simulink model "paper"  (R2022a)
settings: Solver=VariableStepAuto  StartTime=0.0  StopTime=10.0  RelTol=1e-3
values from neighbouring files (symbols this model uses):
  Ce = 0.556    [Untitled.m]    (also in liner.m)
  Ied = 4    [liner.m]
  Ki = 5    [Untitled.m]    (also in liner.m = 1)
  Kn = 7.84    [Untitled.m]    (also in liner.m = 29.75)
  Ks = 1    [Untitled.m]    (also in liner.m)
  ned = 5    [liner.m]
  R = 0.6    [Untitled.m]    (also in liner.m)
  Tl = 0.167    [Untitled.m]    (also in liner.m)
  Tm = 0.282    [Untitled.m]    (also in liner.m)
  Ts = 0.01    [Untitled.m]    (also in liner.m)
undefined symbols (not defined in the file or in its folder): alpha, beta, lambda, tau_i, tau_n, Ud, Ued
settings Model: Creator=houtonglei  LastModifiedBy=houtonglei
settings DataIOCC: SaveFinalState=on  SaveState=on

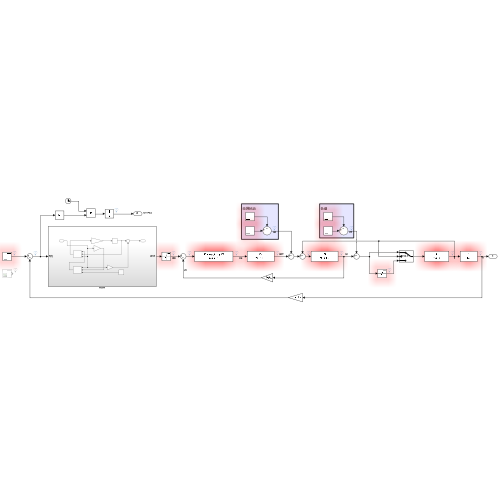
[thumbnail: Simulink's stored preview of the top-level diagram]
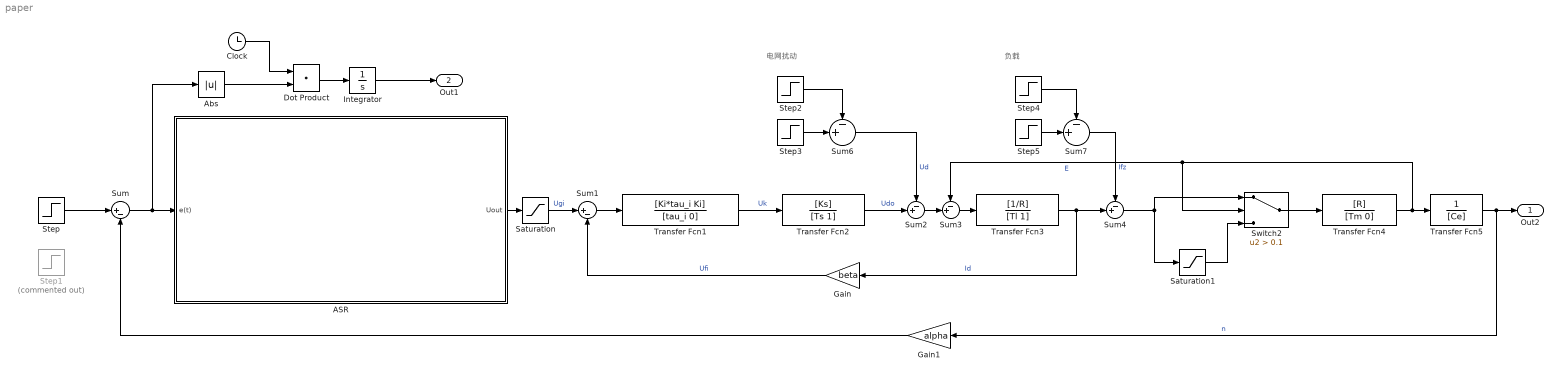
== system paper ==
  note: 负载
  note: 电网扰动
  ASR : Subsystem
  Abs : Abs  SaturateOnIntegerOverflow=off
  Clock : Clock
  Dot Product : DotProduct  OutDataTypeStr=Inherit: Inherit via internal rule
  Gain : Gain  Gain=beta
  Gain1 : Gain  Gain=alpha
  Integrator : Integrator
  Saturation : Saturate  UpperLimit=lambda*Ued  LowerLimit=-lambda*Ued
  Saturation1 : Saturate  UpperLimit=lambda*Ied  LowerLimit=0
  Step : Step  Time=0  After=ned  SampleTime=0
  Step1 : Step  Commented=on  Time=0  After=ned  SampleTime=0
  Step2 : Step  Time=2  After=-0.1*Ud  SampleTime=0
  Step3 : Step  After=-0.1*Ud  SampleTime=0
  Step4 : Step  Time=2  After=0.5*Ied  SampleTime=0
  Step5 : Step  After=0.5*Ied  SampleTime=0
  Sum : Sum  Inputs=|+-
  Sum1 : Sum  Inputs=|+-
  Sum{2..4,6..7} (5 alike) : Sum  Inputs=-+|
  Switch2 : Switch  Criteria=u2 > Threshold  Threshold=0.1  SaturateOnIntegerOverflow=off  InputSameDT=off
  Transfer Fcn1 : TransferFcn  Numerator=[Ki*tau_i Ki]  Denominator=[tau_i 0]  ContinuousStateAttributes='ACR'
  Transfer Fcn2 : TransferFcn  Numerator=[Ks]  Denominator=[Ts 1]  ContinuousStateAttributes='PWM'
  Transfer Fcn3 : TransferFcn  Numerator=[1/R]  Denominator=[Tl 1]
  Transfer Fcn4 : TransferFcn  Numerator=[R]  Denominator=[Tm 0]
  Transfer Fcn5 : TransferFcn  Denominator=[Ce]
  Out2 : Outport
  Out1 : Outport  Port=2  SignalName=J(ITAE)
  wires:
  Saturation/1 -> Sum1/1  "Ugi"
  Gain1/1 -> Sum/2
  Gain/1 -> Sum1/2  "Ufi"
  Transfer Fcn1/1 -> Transfer Fcn2/1  "Uk"
  Sum2/1 -> Sum3/2
  Transfer Fcn4/1 -> Transfer Fcn5/1, Switch2/2, Sum3/1  "E"
  Transfer Fcn5/1 -> Out2/1, Gain1/1  "n"
  Transfer Fcn2/1 -> Sum2/2  "Udo"
  Clock/1 -> Dot Product/1
  Abs/1 -> Dot Product/2
  Dot Product/1 -> Integrator/1
  Sum3/1 -> Transfer Fcn3/1
  Integrator/1 -> Out1/1
  Sum1/1 -> Transfer Fcn1/1
  Sum/1 -> Abs/1, ASR/1(e(t))
  Transfer Fcn3/1 -> Sum4/2, Gain/1  "Id"
  Switch2/1 -> Transfer Fcn4/1
  Saturation1/1 -> Switch2/3
  Sum4/1 -> Switch2/1, Saturation1/1
  Sum7/1 -> Sum4/1  "Ifz"
  Sum6/1 -> Sum2/1  "Ud"
  Step3/1 -> Sum6/2
  Step2/1 -> Sum6/1
  Step5/1 -> Sum7/2
  Step4/1 -> Sum7/1
  ASR/1(Uout) -> Saturation/1
  Step/1 -> Sum/1

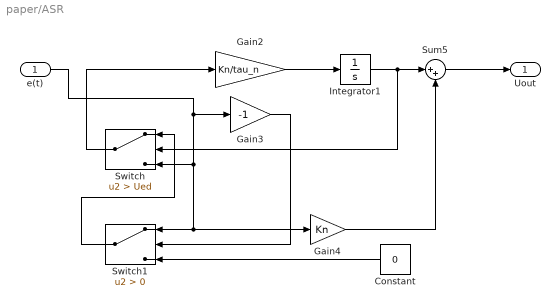
== system paper/ASR ==
  e(t) : Inport
  Constant : Constant  Value=0
  Gain2 : Gain  Gain=Kn/tau_n
  Gain3 : Gain  Gain=-1
  Gain4 : Gain  Gain=Kn
  Integrator1 : Integrator
  Sum5 : Sum  Inputs=|++
  Switch : Switch  Criteria=u2 > Threshold  Threshold=Ued  SaturateOnIntegerOverflow=off  InputSameDT=off
  Switch1 : Switch  Criteria=u2 > Threshold  SaturateOnIntegerOverflow=off  InputSameDT=off
  Uout : Outport
  wires:
  Sum5/1 -> Uout/1
  Switch1/1 -> Switch/1
  Switch/1 -> Gain2/1
  Gain2/1 -> Integrator1/1
  Gain4/1 -> Sum5/2
  Integrator1/1 -> Switch/2, Sum5/1
  Gain3/1 -> Switch1/2
  e(t)/1 -> Gain4/1, Switch1/1, Switch/3, Gain3/1
  Constant/1 -> Switch1/3
